simulink model "pcm_microphone"  (R2018a)
settings: Solver=VariableStepAuto  StartTime=0.0  StopTime=10.0  RelTol=1e-3
libraries: dsparch4 x2, commutil2 x2, dspquant2 x2, audiosources x1, dspsigops x1
settings Model: Creator=hp  LastModifiedBy=hp

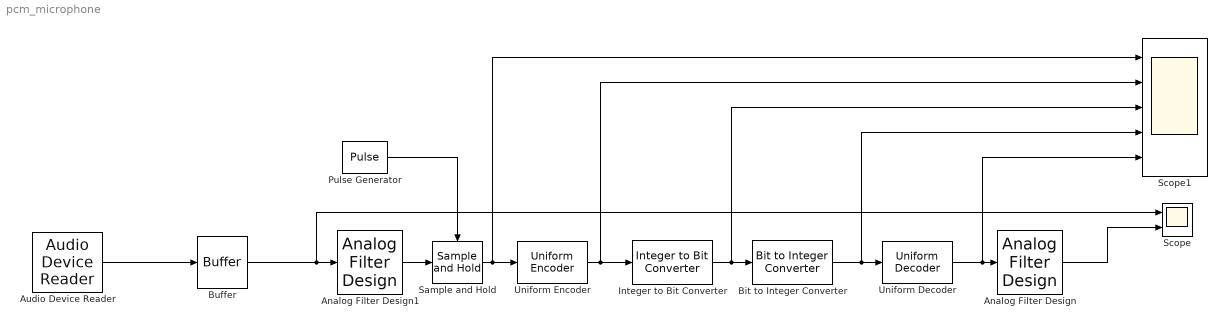
== system pcm_microphone ==
  Analog Filter Design : dsparch4/Analog Filter Design  method=Butterworth  filttype=Bandpass  N=8  Wlo=2*pi*300  Whi=2*pi*3400  Rp=2  Rs=40
  Analog Filter Design1 : dsparch4/Analog Filter Design  method=Butterworth  filttype=Bandpass  N=8  Wlo=2*pi*300  Whi=2*pi*3400  Rp=2  Rs=40
  Audio Device Reader : audiosources/Audio Device Reader  Driver=DirectSound  Device=Default  SampleRate=8000  NumChannels=1  SamplesPerFrame=2  BitDepth=16-bit integer  NumBuffers=10  DefaultInputChannelMapping=on  InputChannelMapping=1:2  OutputNumOverrunSamples=off  OutputDataType=double  DriverIdx=1  DeviceWarnFlag=''
      settings: SourceProductName=Audio System Toolbox  SourceProductBaseCode=AU
  Bit to Integer Converter : commutil2/Bit to Integer Converter  nbits=8  bitOrder=MSB first  signedOutputValues=Unsigned  outDtype=Inherit via internal rule  outDtypeSigned=Inherit via internal rule
  Buffer : Buffer  N=1  OutputFrames=off
  Integer to Bit Converter : commutil2/Integer to Bit Converter  nbits=8  signedInputValues=Unsigned  bitOrder=MSB first  outDtype=Inherit via internal rule
  Pulse Generator : DiscretePulseGenerator  PulseType=Time based  Period=1/8000  PulseWidth=50
  Sample and Hold : dspsigops/Sample and Hold  trig=Rising edge  initCond=0  latchinput=off
  Scope : Scope  NumInputPorts=2
  Scope1 : Scope  NumInputPorts=5
  Uniform Decoder : dspquant2/Uniform Decoder  peak=1  bits=8  overflowMode=Saturate  otype=Double
      settings: SourceProductName=DSP System Toolbox  SourceProductBaseCode=DS
  Uniform Encoder : dspquant2/Uniform Encoder  peak=1  bits=8  otype=Unsigned integer
      settings: SourceProductName=DSP System Toolbox
  wires:
  Pulse Generator/1 -> Sample and Hold/Trigger
  Buffer/1 -> Scope/1, Analog Filter Design1/1
  Integer to Bit Converter/1 -> Scope1/3, Bit to Integer Converter/1
  Analog Filter Design1/1 -> Sample and Hold/1
  Bit to Integer Converter/1 -> Scope1/4, Uniform Decoder/1
  Analog Filter Design/1 -> Scope/2
  Uniform Encoder/1 -> Scope1/2, Integer to Bit Converter/1
  Uniform Decoder/1 -> Scope1/5, Analog Filter Design/1
  Sample and Hold/1 -> Scope1/1, Uniform Encoder/1
  Audio Device Reader/1 -> Buffer/1
